simulink library "halout"  (R2021b)
settings: Solver=VariableStepAuto  StartTime=0.0  StopTime=10.0  RelTol=1e-3
undefined symbols (not defined in the file): C_TASK_5MS_S, FALSE, KHAL_CAN1TxReq_flg, KHAL_CAN2TxReq_flg, KHAL_CAN3FD3VCU1toNIDECTxReq_flg, KHAL_CAN3FD3VCU1TxReq_flg, KHAL_CAN3FD3VCU2E2E_flg, KHAL_CAN3FD3VCU2toNIDECE2E_flg, KHAL_CAN3FD3VCU2toNIDECTxReq_flg, KHAL_CAN3FD3VCU2TxReq_flg, KHAL_CAN3TxReq_flg, KHAL_CAN4FD4CE1000E2E_flg, KHAL_CAN4FD4CE1000TxReq_flg, KHAL_CAN4TxReq_flg, KHAL_CAN5TxReq_flg, KHAL_CAN7TxReq_flg, ONE_INT, TRUE, ZERO_INT
libraries: FVT_lib x258, simulink x115
(part 4 of 17)

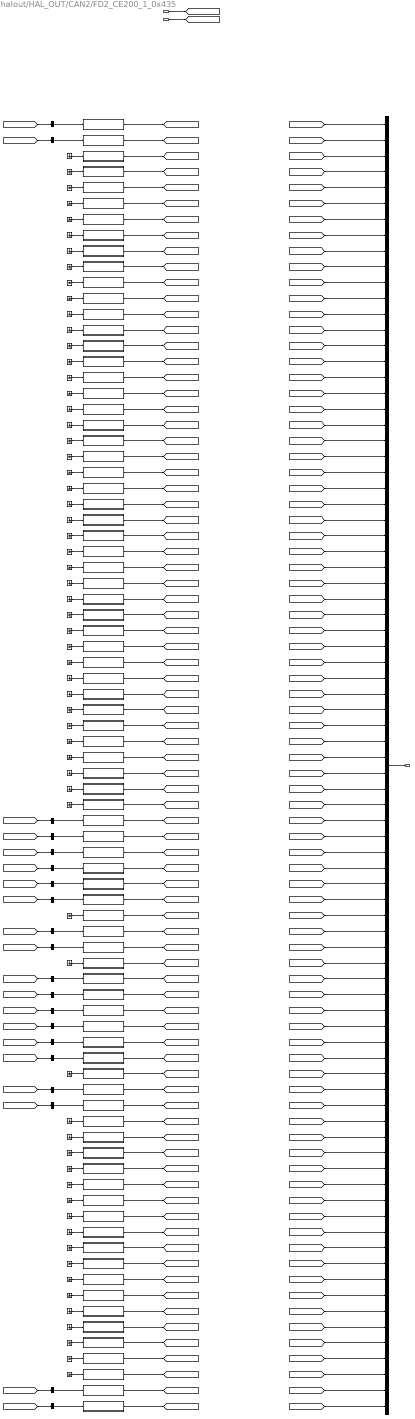
== system halout/HAL_OUT/CAN2/FD2_CE200_1_0x435 ==
  BSCP_outputs : Inport  OutDataTypeStr=Bus: BSCP_outputs
  BOUTP_outputs : Inport  Port=2  OutDataTypeStr=Bus: BOUTP_outputs
  AutoLTips : Subsystem
  CWheelTips : Subsystem
  FDCBCMAcc1StaSta : Subsystem
  FDCBCMAcc2StaSta : Subsystem
  FDCBCMAcc3StaSta : Subsystem
  FDCBCMAcc4StaSta : Subsystem
  FDCBCMAcc5StaSta : Subsystem
  FDCBCMAmbBrightStaSta : Subsystem
  FDCBCMAmbColorStaSta : Subsystem
  FDCBCMAmbDimENSta : Subsystem
  FDCBCMAmbFunENSta : Subsystem
  FDCBCMAmbLinkDriStaSta : Subsystem
  FDCBCMAmbODAENSta : Subsystem
  FDCBCMAmbPwrWarnENSta : Subsystem
  FDCBCMAmbWelENSta : Subsystem
  FDCBCMCLWinLockDrSta : Subsystem
  FDCBCMFollowMeENFunSta : Subsystem
  FDCBCMKey10AccSta : Subsystem
  FDCBCMKey1AccSta : Subsystem
  FDCBCMKey2AccSta : Subsystem
  FDCBCMKey3AccSta : Subsystem
  FDCBCMKey4AccSta : Subsystem
  FDCBCMKey5AccSta : Subsystem
  FDCBCMKey6AccSta : Subsystem
  FDCBCMKey7AccSta : Subsystem
  FDCBCMKey8AccSta : Subsystem
  FDCBCMKey9AccSta : Subsystem
  FDCBCMLockAlarmCmd : Subsystem
  FDCBCMPTGOpenHeightSta : Subsystem
  FDCBCMRmLpModeENFunSta : Subsystem
  FDCBCMTurnSwTSetStaSta : Subsystem
  FDCBCMUserNowSta : Subsystem
  FDCBCMWalkInUnLkEnFunSta : Subsystem
  FDCBCMWalkOutLkEnFunSta : Subsystem
  FDCDKCDkeyShowIVISta : Subsystem
  FDCDKCKeyMissSta : Subsystem
  FDCDKCKeyNumSta : Subsystem
  FDCDKCKeyTypeSta : Subsystem
  FDCDKCUIDLowPowerSta : Subsystem
  FDCSPTGSPTGENFunSta : Subsystem
  FDCTHCMAPTCForceOFFSta : Subsystem
  FDCTHCMAPTCWarningSta : Subsystem
  FDCTHCMAirIntZ3Sta : Subsystem
  Ground{,1..61} (62 alike) : Ground
  LFWheelShield : Subsystem
  LRBatWarn : Subsystem
  LRPressIndi : Subsystem
  LRSensorFail : Subsystem
  LRWheelDebug : Subsystem
  LRWheelPSW : Subsystem
  LRWheelPress : Subsystem
  LRWheelShield : Subsystem
  LRWheelTemp : Subsystem
  LRWheelTmpIndi : Subsystem
  RFWheelShield : Subsystem
  RRBatWarn : Subsystem
  RRPressIndi : Subsystem
  RRSensorFail : Subsystem
  RRWheelDebug : Subsystem
  RRWheelPSW : Subsystem
  RRWheelPress : Subsystem
  RRWheelShield : Subsystem
  RRWheelTemp : Subsystem
  RRWheelTmpIndi : Subsystem
  T1TPMSLFBatWarn : Subsystem
  T1TPMSLFPressIndi : Subsystem
  T1TPMSLFSensorFail : Subsystem
  T1TPMSLFWheelDebug : Subsystem
  T1TPMSLFWheelPSW : Subsystem
  T1TPMSLFWheelPress : Subsystem
  T1TPMSLFWheelTemp : Subsystem
  T1TPMSLFWheelTmpIndi : Subsystem
  T1TPMSRFBatWarn : Subsystem
  T1TPMSRFPressIndi : Subsystem
  T1TPMSRFSensorFail : Subsystem
  T1TPMSRFWheelDebug : Subsystem
  T1TPMSRFWheelPSW : Subsystem
  T1TPMSRFWheelPress : Subsystem
  T1TPMSRFWheelTemp : Subsystem
  T1TPMSRFWheelTmpIndi : Subsystem
  T1TPMSTPMSWarnIndi : Subsystem
  TPMSCaliButtAllow : Subsystem
  TPMSResButtAllow : Subsystem
  bus_creator : BusCreator  Inputs=82  OutDataTypeStr=Bus: DT_CAN2_SG_FD2_CE200_1  NonVirtualBus=on
  bus_selector : BusSelector  OutputSignals=VOUTP_AutoLTips_enum
  bus_selector1 : BusSelector  OutputSignals=VOUTP_CWheelTips_enum
  bus_selector10 : BusSelector  OutputSignals=VOUTP_RRBatWarn_flg
  bus_selector11 : BusSelector  OutputSignals=VOUTP_RRPressIndi_enum
  bus_selector12 : BusSelector  OutputSignals=VOUTP_RRSensorFail_flg
  bus_selector13 : BusSelector  OutputSignals=VOUTP_RRWheelDebug_flg
  bus_selector14 : BusSelector  OutputSignals=VOUTP_RRWheelPSW_raw8
  bus_selector15 : BusSelector  OutputSignals=VOUTP_RRWheelPress_raw8
  bus_selector16 : BusSelector  OutputSignals=VOUTP_RRWheelTemp_C
  bus_selector17 : BusSelector  OutputSignals=VOUTP_RRWheelTmpIndi_flg
  bus_selector18 : BusSelector  OutputSignals=VOUTP_TPMSCaliButtAllow_flg
  bus_selector19 : BusSelector  OutputSignals=VOUTP_TPMSResButtAllow_flg
  bus_selector2 : BusSelector  OutputSignals=VOUTP_LRBatWarn_flg
  bus_selector3 : BusSelector  OutputSignals=VOUTP_LRPressIndi_enum
  bus_selector4 : BusSelector  OutputSignals=VOUTP_LRSensorFail_flg
  bus_selector5 : BusSelector  OutputSignals=VOUTP_LRWheelDebug_flg
  bus_selector6 : BusSelector  OutputSignals=VOUTP_LRWheelPSW_raw8
  bus_selector7 : BusSelector  OutputSignals=VOUTP_LRWheelPress_raw8
  bus_selector8 : BusSelector  OutputSignals=VOUTP_LRWheelTemp_C
  bus_selector9 : BusSelector  OutputSignals=VOUTP_LRWheelTmpIndi_flg
  FD2_CE200_1 : Outport
  wires:
  BSCP_outputs/1 -> [BSCP_outputs]
  BOUTP_outputs/1 -> [BOUTP_outputs]
  [CAN2_AutoLTips] -> bus_creator/1  "CAN2_AutoLTips"
  [CAN2_CWheelTips] -> bus_creator/2  "CAN2_CWheelTips"
  [CAN2_FDC_BCM_Acc1Sta_Sta] -> bus_creator/3  "CAN2_FDC_BCM_Acc1Sta_Sta"
  [CAN2_FDC_BCM_Acc2Sta_Sta] -> bus_creator/4  "CAN2_FDC_BCM_Acc2Sta_Sta"
  [CAN2_FDC_BCM_Acc3Sta_Sta] -> bus_creator/5  "CAN2_FDC_BCM_Acc3Sta_Sta"
  [CAN2_FDC_BCM_Acc4Sta_Sta] -> bus_creator/6  "CAN2_FDC_BCM_Acc4Sta_Sta"
  [CAN2_FDC_BCM_Acc5Sta_Sta] -> bus_creator/7  "CAN2_FDC_BCM_Acc5Sta_Sta"
  [CAN2_FDC_BCM_AmbBrightSta_Sta] -> bus_creator/8  "CAN2_FDC_BCM_AmbBrightSta_Sta"
  [CAN2_FDC_BCM_AmbColorSta_Sta] -> bus_creator/9  "CAN2_FDC_BCM_AmbColorSta_Sta"
  [CAN2_FDC_BCM_AmbDimEN_Sta] -> bus_creator/10  "CAN2_FDC_BCM_AmbDimEN_Sta"
  [CAN2_FDC_BCM_AmbFunEN_Sta] -> bus_creator/11  "CAN2_FDC_BCM_AmbFunEN_Sta"
  [CAN2_FDC_BCM_AmbLinkDriSta_Sta] -> bus_creator/12  "CAN2_FDC_BCM_AmbLinkDriSta_Sta"
  [CAN2_FDC_BCM_AmbODAEN_Sta] -> bus_creator/13  "CAN2_FDC_BCM_AmbODAEN_Sta"
  [CAN2_FDC_BCM_AmbPwrWarnEN_Sta] -> bus_creator/14  "CAN2_FDC_BCM_AmbPwrWarnEN_Sta"
  [CAN2_FDC_BCM_AmbWelEN_Sta] -> bus_creator/15  "CAN2_FDC_BCM_AmbWelEN_Sta"
  [CAN2_FDC_BCM_CLWinLockDr_Sta] -> bus_creator/16  "CAN2_FDC_BCM_CLWinLockDr_Sta"
  [CAN2_FDC_BCM_FollowMeENFun_Sta] -> bus_creator/17  "CAN2_FDC_BCM_FollowMeENFun_Sta"
  [CAN2_FDC_BCM_Key10Acc_Sta] -> bus_creator/18  "CAN2_FDC_BCM_Key10Acc_Sta"
  [CAN2_FDC_BCM_Key1Acc_Sta] -> bus_creator/19  "CAN2_FDC_BCM_Key1Acc_Sta"
  [CAN2_FDC_BCM_Key2Acc_Sta] -> bus_creator/20  "CAN2_FDC_BCM_Key2Acc_Sta"
  [CAN2_FDC_BCM_Key3Acc_Sta] -> bus_creator/21  "CAN2_FDC_BCM_Key3Acc_Sta"
  [CAN2_FDC_BCM_Key4Acc_Sta] -> bus_creator/22  "CAN2_FDC_BCM_Key4Acc_Sta"
  [CAN2_FDC_BCM_Key5Acc_Sta] -> bus_creator/23  "CAN2_FDC_BCM_Key5Acc_Sta"
  [CAN2_FDC_BCM_Key6Acc_Sta] -> bus_creator/24  "CAN2_FDC_BCM_Key6Acc_Sta"
  [CAN2_FDC_BCM_Key7Acc_Sta] -> bus_creator/25  "CAN2_FDC_BCM_Key7Acc_Sta"
  [CAN2_FDC_BCM_Key8Acc_Sta] -> bus_creator/26  "CAN2_FDC_BCM_Key8Acc_Sta"
  [CAN2_FDC_BCM_Key9Acc_Sta] -> bus_creator/27  "CAN2_FDC_BCM_Key9Acc_Sta"
  [CAN2_FDC_BCM_LockAlarm_Cmd] -> bus_creator/28  "CAN2_FDC_BCM_LockAlarm_Cmd"
  [CAN2_FDC_BCM_PTGOpenHeight_Sta] -> bus_creator/29  "CAN2_FDC_BCM_PTGOpenHeight_Sta"
  [CAN2_FDC_BCM_RmLpModeENFun_Sta] -> bus_creator/30  "CAN2_FDC_BCM_RmLpModeENFun_Sta"
  [CAN2_FDC_BCM_TurnSwTSetSta_Sta] -> bus_creator/31  "CAN2_FDC_BCM_TurnSwTSetSta_Sta"
  [CAN2_FDC_BCM_UserNow_Sta] -> bus_creator/32  "CAN2_FDC_BCM_UserNow_Sta"
  [CAN2_FDC_BCM_WalkInUnLkEnFun_Sta] -> bus_creator/33  "CAN2_FDC_BCM_WalkInUnLkEnFun_Sta"
  [CAN2_FDC_BCM_WalkOutLkEnFun_Sta] -> bus_creator/34  "CAN2_FDC_BCM_WalkOutLkEnFun_Sta"
  [CAN2_FDC_DKC_DkeyShowIVI_Sta] -> bus_creator/35  "CAN2_FDC_DKC_DkeyShowIVI_Sta"
  [CAN2_FDC_DKC_KeyMiss_Sta] -> bus_creator/36  "CAN2_FDC_DKC_KeyMiss_Sta"
  [CAN2_FDC_DKC_KeyNum_Sta] -> bus_creator/37  "CAN2_FDC_DKC_KeyNum_Sta"
  [CAN2_FDC_DKC_KeyType_Sta] -> bus_creator/38  "CAN2_FDC_DKC_KeyType_Sta"
  [CAN2_FDC_DKC_UIDLowPower_Sta] -> bus_creator/39  "CAN2_FDC_DKC_UIDLowPower_Sta"
  [CAN2_FDC_SPTG_SPTGENFun_Sta] -> bus_creator/40  "CAN2_FDC_SPTG_SPTGENFun_Sta"
  [CAN2_FDC_THCM_APTCForceOFF_Sta] -> bus_creator/41  "CAN2_FDC_THCM_APTCForceOFF_Sta"
  [CAN2_FDC_THCM_APTCWarning_Sta] -> bus_creator/42  "CAN2_FDC_THCM_APTCWarning_Sta"
  [CAN2_FDC_THCM_AirIntZ3_Sta] -> bus_creator/43  "CAN2_FDC_THCM_AirIntZ3_Sta"
  [CAN2_LFWheelShield] -> bus_creator/44  "CAN2_LFWheelShield"
  [CAN2_LRBatWarn] -> bus_creator/45  "CAN2_LRBatWarn"
  [CAN2_LRPressIndi] -> bus_creator/46  "CAN2_LRPressIndi"
  [CAN2_LRSensorFail] -> bus_creator/47  "CAN2_LRSensorFail"
  [CAN2_LRWheelDebug] -> bus_creator/48  "CAN2_LRWheelDebug"
  [CAN2_LRWheelPSW] -> bus_creator/49  "CAN2_LRWheelPSW"
  [CAN2_LRWheelPress] -> bus_creator/50  "CAN2_LRWheelPress"
  [CAN2_LRWheelShield] -> bus_creator/51  "CAN2_LRWheelShield"
  [CAN2_LRWheelTemp] -> bus_creator/52  "CAN2_LRWheelTemp"
  [CAN2_LRWheelTmpIndi] -> bus_creator/53  "CAN2_LRWheelTmpIndi"
  [CAN2_RFWheelShield] -> bus_creator/54  "CAN2_RFWheelShield"
  [CAN2_RRBatWarn] -> bus_creator/55  "CAN2_RRBatWarn"
  [CAN2_RRPressIndi] -> bus_creator/56  "CAN2_RRPressIndi"
  [CAN2_RRSensorFail] -> bus_creator/57  "CAN2_RRSensorFail"
  [CAN2_RRWheelDebug] -> bus_creator/58  "CAN2_RRWheelDebug"
  [CAN2_RRWheelPSW] -> bus_creator/59  "CAN2_RRWheelPSW"
  [CAN2_RRWheelPress] -> bus_creator/60  "CAN2_RRWheelPress"
  [CAN2_RRWheelShield] -> bus_creator/61  "CAN2_RRWheelShield"
  [CAN2_RRWheelTemp] -> bus_creator/62  "CAN2_RRWheelTemp"
  [CAN2_RRWheelTmpIndi] -> bus_creator/63  "CAN2_RRWheelTmpIndi"
  [CAN2_T1_TPMS_LFBatWarn] -> bus_creator/64  "CAN2_T1_TPMS_LFBatWarn"
  [CAN2_T1_TPMS_LFPressIndi] -> bus_creator/65  "CAN2_T1_TPMS_LFPressIndi"
  [CAN2_T1_TPMS_LFSensorFail] -> bus_creator/66  "CAN2_T1_TPMS_LFSensorFail"
  [CAN2_T1_TPMS_LFWheelDebug] -> bus_creator/67  "CAN2_T1_TPMS_LFWheelDebug"
  [CAN2_T1_TPMS_LFWheelPSW] -> bus_creator/68  "CAN2_T1_TPMS_LFWheelPSW"
  [CAN2_T1_TPMS_LFWheelPress] -> bus_creator/69  "CAN2_T1_TPMS_LFWheelPress"
  [CAN2_T1_TPMS_LFWheelTemp] -> bus_creator/70  "CAN2_T1_TPMS_LFWheelTemp"
  [CAN2_T1_TPMS_LFWheelTmpIndi] -> bus_creator/71  "CAN2_T1_TPMS_LFWheelTmpIndi"
  [CAN2_T1_TPMS_RFBatWarn] -> bus_creator/72  "CAN2_T1_TPMS_RFBatWarn"
  [CAN2_T1_TPMS_RFPressIndi] -> bus_creator/73  "CAN2_T1_TPMS_RFPressIndi"
  [CAN2_T1_TPMS_RFSensorFail] -> bus_creator/74  "CAN2_T1_TPMS_RFSensorFail"
  [CAN2_T1_TPMS_RFWheelDebug] -> bus_creator/75  "CAN2_T1_TPMS_RFWheelDebug"
  [CAN2_T1_TPMS_RFWheelPSW] -> bus_creator/76  "CAN2_T1_TPMS_RFWheelPSW"
  [CAN2_T1_TPMS_RFWheelPress] -> bus_creator/77  "CAN2_T1_TPMS_RFWheelPress"
  [CAN2_T1_TPMS_RFWheelTemp] -> bus_creator/78  "CAN2_T1_TPMS_RFWheelTemp"
  [CAN2_T1_TPMS_RFWheelTmpIndi] -> bus_creator/79  "CAN2_T1_TPMS_RFWheelTmpIndi"
  [CAN2_T1_TPMS_TPMSWarnIndi] -> bus_creator/80  "CAN2_T1_TPMS_TPMSWarnIndi"
  [CAN2_TPMS_Cali_Butt_Allow] -> bus_creator/81  "CAN2_TPMS_Cali_Butt_Allow"
  [CAN2_TPMS_Res_Butt_Allow] -> bus_creator/82  "CAN2_TPMS_Res_Butt_Allow"
  bus_creator/1 -> FD2_CE200_1/1
  AutoLTips/1(CAN2_AutoLTips) -> [CAN2_AutoLTips]
  CWheelTips/1(CAN2_CWheelTips) -> [CAN2_CWheelTips]
  FDCBCMAcc1StaSta/1(CAN2_FDC_BCM_Acc1Sta_Sta) -> [CAN2_FDC_BCM_Acc1Sta_Sta]
  FDCBCMAcc2StaSta/1(CAN2_FDC_BCM_Acc2Sta_Sta) -> [CAN2_FDC_BCM_Acc2Sta_Sta]
  FDCBCMAcc3StaSta/1(CAN2_FDC_BCM_Acc3Sta_Sta) -> [CAN2_FDC_BCM_Acc3Sta_Sta]
  FDCBCMAcc4StaSta/1(CAN2_FDC_BCM_Acc4Sta_Sta) -> [CAN2_FDC_BCM_Acc4Sta_Sta]
  FDCBCMAcc5StaSta/1(CAN2_FDC_BCM_Acc5Sta_Sta) -> [CAN2_FDC_BCM_Acc5Sta_Sta]
  FDCBCMAmbBrightStaSta/1(CAN2_FDC_BCM_AmbBrightSta_Sta) -> [CAN2_FDC_BCM_AmbBrightSta_Sta]
  FDCBCMAmbColorStaSta/1(CAN2_FDC_BCM_AmbColorSta_Sta) -> [CAN2_FDC_BCM_AmbColorSta_Sta]
  FDCBCMAmbDimENSta/1(CAN2_FDC_BCM_AmbDimEN_Sta) -> [CAN2_FDC_BCM_AmbDimEN_Sta]
  FDCBCMAmbFunENSta/1(CAN2_FDC_BCM_AmbFunEN_Sta) -> [CAN2_FDC_BCM_AmbFunEN_Sta]
  FDCBCMAmbLinkDriStaSta/1(CAN2_FDC_BCM_AmbLinkDriSta_Sta) -> [CAN2_FDC_BCM_AmbLinkDriSta_Sta]
  FDCBCMAmbODAENSta/1(CAN2_FDC_BCM_AmbODAEN_Sta) -> [CAN2_FDC_BCM_AmbODAEN_Sta]
  FDCBCMAmbPwrWarnENSta/1(CAN2_FDC_BCM_AmbPwrWarnEN_Sta) -> [CAN2_FDC_BCM_AmbPwrWarnEN_Sta]
  FDCBCMAmbWelENSta/1(CAN2_FDC_BCM_AmbWelEN_Sta) -> [CAN2_FDC_BCM_AmbWelEN_Sta]
  FDCBCMCLWinLockDrSta/1(CAN2_FDC_BCM_CLWinLockDr_Sta) -> [CAN2_FDC_BCM_CLWinLockDr_Sta]
  FDCBCMFollowMeENFunSta/1(CAN2_FDC_BCM_FollowMeENFun_Sta) -> [CAN2_FDC_BCM_FollowMeENFun_Sta]
  FDCBCMKey10AccSta/1(CAN2_FDC_BCM_Key10Acc_Sta) -> [CAN2_FDC_BCM_Key10Acc_Sta]
  FDCBCMKey1AccSta/1(CAN2_FDC_BCM_Key1Acc_Sta) -> [CAN2_FDC_BCM_Key1Acc_Sta]
  FDCBCMKey2AccSta/1(CAN2_FDC_BCM_Key2Acc_Sta) -> [CAN2_FDC_BCM_Key2Acc_Sta]
  FDCBCMKey3AccSta/1(CAN2_FDC_BCM_Key3Acc_Sta) -> [CAN2_FDC_BCM_Key3Acc_Sta]
  FDCBCMKey4AccSta/1(CAN2_FDC_BCM_Key4Acc_Sta) -> [CAN2_FDC_BCM_Key4Acc_Sta]
  FDCBCMKey5AccSta/1(CAN2_FDC_BCM_Key5Acc_Sta) -> [CAN2_FDC_BCM_Key5Acc_Sta]
  FDCBCMKey6AccSta/1(CAN2_FDC_BCM_Key6Acc_Sta) -> [CAN2_FDC_BCM_Key6Acc_Sta]
  FDCBCMKey7AccSta/1(CAN2_FDC_BCM_Key7Acc_Sta) -> [CAN2_FDC_BCM_Key7Acc_Sta]
  FDCBCMKey8AccSta/1(CAN2_FDC_BCM_Key8Acc_Sta) -> [CAN2_FDC_BCM_Key8Acc_Sta]
  FDCBCMKey9AccSta/1(CAN2_FDC_BCM_Key9Acc_Sta) -> [CAN2_FDC_BCM_Key9Acc_Sta]
  FDCBCMLockAlarmCmd/1(CAN2_FDC_BCM_LockAlarm_Cmd) -> [CAN2_FDC_BCM_LockAlarm_Cmd]
  FDCBCMPTGOpenHeightSta/1(CAN2_FDC_BCM_PTGOpenHeight_Sta) -> [CAN2_FDC_BCM_PTGOpenHeight_Sta]
  FDCBCMRmLpModeENFunSta/1(CAN2_FDC_BCM_RmLpModeENFun_Sta) -> [CAN2_FDC_BCM_RmLpModeENFun_Sta]
  FDCBCMTurnSwTSetStaSta/1(CAN2_FDC_BCM_TurnSwTSetSta_Sta) -> [CAN2_FDC_BCM_TurnSwTSetSta_Sta]
  FDCBCMUserNowSta/1(CAN2_FDC_BCM_UserNow_Sta) -> [CAN2_FDC_BCM_UserNow_Sta]
  FDCBCMWalkInUnLkEnFunSta/1(CAN2_FDC_BCM_WalkInUnLkEnFun_Sta) -> [CAN2_FDC_BCM_WalkInUnLkEnFun_Sta]
  FDCBCMWalkOutLkEnFunSta/1(CAN2_FDC_BCM_WalkOutLkEnFun_Sta) -> [CAN2_FDC_BCM_WalkOutLkEnFun_Sta]
  FDCDKCDkeyShowIVISta/1(CAN2_FDC_DKC_DkeyShowIVI_Sta) -> [CAN2_FDC_DKC_DkeyShowIVI_Sta]
  FDCDKCKeyMissSta/1(CAN2_FDC_DKC_KeyMiss_Sta) -> [CAN2_FDC_DKC_KeyMiss_Sta]
  FDCDKCKeyNumSta/1(CAN2_FDC_DKC_KeyNum_Sta) -> [CAN2_FDC_DKC_KeyNum_Sta]
  FDCDKCKeyTypeSta/1(CAN2_FDC_DKC_KeyType_Sta) -> [CAN2_FDC_DKC_KeyType_Sta]
  FDCDKCUIDLowPowerSta/1(CAN2_FDC_DKC_UIDLowPower_Sta) -> [CAN2_FDC_DKC_UIDLowPower_Sta]
  FDCSPTGSPTGENFunSta/1(CAN2_FDC_SPTG_SPTGENFun_Sta) -> [CAN2_FDC_SPTG_SPTGENFun_Sta]
  FDCTHCMAPTCForceOFFSta/1(CAN2_FDC_THCM_APTCForceOFF_Sta) -> [CAN2_FDC_THCM_APTCForceOFF_Sta]
  FDCTHCMAPTCWarningSta/1(CAN2_FDC_THCM_APTCWarning_Sta) -> [CAN2_FDC_THCM_APTCWarning_Sta]
  FDCTHCMAirIntZ3Sta/1(CAN2_FDC_THCM_AirIntZ3_Sta) -> [CAN2_FDC_THCM_AirIntZ3_Sta]
  LFWheelShield/1(CAN2_LFWheelShield) -> [CAN2_LFWheelShield]
  LRBatWarn/1(CAN2_LRBatWarn) -> [CAN2_LRBatWarn]
  LRPressIndi/1(CAN2_LRPressIndi) -> [CAN2_LRPressIndi]
  LRSensorFail/1(CAN2_LRSensorFail) -> [CAN2_LRSensorFail]
  LRWheelDebug/1(CAN2_LRWheelDebug) -> [CAN2_LRWheelDebug]
  LRWheelPSW/1(CAN2_LRWheelPSW) -> [CAN2_LRWheelPSW]
  LRWheelPress/1(CAN2_LRWheelPress) -> [CAN2_LRWheelPress]
  LRWheelShield/1(CAN2_LRWheelShield) -> [CAN2_LRWheelShield]
  LRWheelTemp/1(CAN2_LRWheelTemp) -> [CAN2_LRWheelTemp]
  LRWheelTmpIndi/1(CAN2_LRWheelTmpIndi) -> [CAN2_LRWheelTmpIndi]
  RFWheelShield/1(CAN2_RFWheelShield) -> [CAN2_RFWheelShield]
  RRBatWarn/1(CAN2_RRBatWarn) -> [CAN2_RRBatWarn]
  RRPressIndi/1(CAN2_RRPressIndi) -> [CAN2_RRPressIndi]
  RRSensorFail/1(CAN2_RRSensorFail) -> [CAN2_RRSensorFail]
  RRWheelDebug/1(CAN2_RRWheelDebug) -> [CAN2_RRWheelDebug]
  RRWheelPSW/1(CAN2_RRWheelPSW) -> [CAN2_RRWheelPSW]
  RRWheelPress/1(CAN2_RRWheelPress) -> [CAN2_RRWheelPress]
  RRWheelShield/1(CAN2_RRWheelShield) -> [CAN2_RRWheelShield]
  RRWheelTemp/1(CAN2_RRWheelTemp) -> [CAN2_RRWheelTemp]
  RRWheelTmpIndi/1(CAN2_RRWheelTmpIndi) -> [CAN2_RRWheelTmpIndi]
  T1TPMSLFBatWarn/1(CAN2_T1_TPMS_LFBatWarn) -> [CAN2_T1_TPMS_LFBatWarn]
  T1TPMSLFPressIndi/1(CAN2_T1_TPMS_LFPressIndi) -> [CAN2_T1_TPMS_LFPressIndi]
  T1TPMSLFSensorFail/1(CAN2_T1_TPMS_LFSensorFail) -> [CAN2_T1_TPMS_LFSensorFail]
  T1TPMSLFWheelDebug/1(CAN2_T1_TPMS_LFWheelDebug) -> [CAN2_T1_TPMS_LFWheelDebug]
  T1TPMSLFWheelPSW/1(CAN2_T1_TPMS_LFWheelPSW) -> [CAN2_T1_TPMS_LFWheelPSW]
  T1TPMSLFWheelPress/1(CAN2_T1_TPMS_LFWheelPress) -> [CAN2_T1_TPMS_LFWheelPress]
  T1TPMSLFWheelTemp/1(CAN2_T1_TPMS_LFWheelTemp) -> [CAN2_T1_TPMS_LFWheelTemp]
  T1TPMSLFWheelTmpIndi/1(CAN2_T1_TPMS_LFWheelTmpIndi) -> [CAN2_T1_TPMS_LFWheelTmpIndi]
  T1TPMSRFBatWarn/1(CAN2_T1_TPMS_RFBatWarn) -> [CAN2_T1_TPMS_RFBatWarn]
  T1TPMSRFPressIndi/1(CAN2_T1_TPMS_RFPressIndi) -> [CAN2_T1_TPMS_RFPressIndi]
  T1TPMSRFSensorFail/1(CAN2_T1_TPMS_RFSensorFail) -> [CAN2_T1_TPMS_RFSensorFail]
  T1TPMSRFWheelDebug/1(CAN2_T1_TPMS_RFWheelDebug) -> [CAN2_T1_TPMS_RFWheelDebug]
  T1TPMSRFWheelPSW/1(CAN2_T1_TPMS_RFWheelPSW) -> [CAN2_T1_TPMS_RFWheelPSW]
  T1TPMSRFWheelPress/1(CAN2_T1_TPMS_RFWheelPress) -> [CAN2_T1_TPMS_RFWheelPress]
  T1TPMSRFWheelTemp/1(CAN2_T1_TPMS_RFWheelTemp) -> [CAN2_T1_TPMS_RFWheelTemp]
  T1TPMSRFWheelTmpIndi/1(CAN2_T1_TPMS_RFWheelTmpIndi) -> [CAN2_T1_TPMS_RFWheelTmpIndi]
  T1TPMSTPMSWarnIndi/1(CAN2_T1_TPMS_TPMSWarnIndi) -> [CAN2_T1_TPMS_TPMSWarnIndi]
  TPMSCaliButtAllow/1(CAN2_TPMS_Cali_Butt_Allow) -> [CAN2_TPMS_Cali_Butt_Allow]
  TPMSResButtAllow/1(CAN2_TPMS_Res_Butt_Allow) -> [CAN2_TPMS_Res_Butt_Allow]
  bus_selector/1 -> AutoLTips/1(AutoLTips)  "<VOUTP_AutoLTips_enum>"
  [BOUTP_outputs] -> bus_selector/1
  bus_selector1/1 -> CWheelTips/1(CWheelTips)  "<VOUTP_CWheelTips_enum>"
  [BOUTP_outputs] -> bus_selector1/1
  Ground/1 -> FDCBCMAcc1StaSta/1(FDCBCMAcc1StaSta)
  Ground1/1 -> FDCBCMAcc2StaSta/1(FDCBCMAcc2StaSta)
  Ground2/1 -> FDCBCMAcc3StaSta/1(FDCBCMAcc3StaSta)
  Ground3/1 -> FDCBCMAcc4StaSta/1(FDCBCMAcc4StaSta)
  Ground4/1 -> FDCBCMAcc5StaSta/1(FDCBCMAcc5StaSta)
  Ground5/1 -> FDCBCMAmbBrightStaSta/1(FDCBCMAmbBrightStaSta)
  Ground6/1 -> FDCBCMAmbColorStaSta/1(FDCBCMAmbColorStaSta)
  Ground7/1 -> FDCBCMAmbDimENSta/1(FDCBCMAmbDimENSta)
  Ground8/1 -> FDCBCMAmbFunENSta/1(FDCBCMAmbFunENSta)
  Ground9/1 -> FDCBCMAmbLinkDriStaSta/1(FDCBCMAmbLinkDriStaSta)
  Ground10/1 -> FDCBCMAmbODAENSta/1(FDCBCMAmbODAENSta)
  Ground11/1 -> FDCBCMAmbPwrWarnENSta/1(FDCBCMAmbPwrWarnENSta)
  Ground12/1 -> FDCBCMAmbWelENSta/1(FDCBCMAmbWelENSta)
  Ground13/1 -> FDCBCMCLWinLockDrSta/1(FDCBCMCLWinLockDrSta)
  Ground14/1 -> FDCBCMFollowMeENFunSta/1(FDCBCMFollowMeENFunSta)
  Ground15/1 -> FDCBCMKey10AccSta/1(FDCBCMKey10AccSta)
  Ground16/1 -> FDCBCMKey1AccSta/1(FDCBCMKey1AccSta)
  Ground17/1 -> FDCBCMKey2AccSta/1(FDCBCMKey2AccSta)
  Ground18/1 -> FDCBCMKey3AccSta/1(FDCBCMKey3AccSta)
  Ground19/1 -> FDCBCMKey4AccSta/1(FDCBCMKey4AccSta)
  Ground20/1 -> FDCBCMKey5AccSta/1(FDCBCMKey5AccSta)
  Ground21/1 -> FDCBCMKey6AccSta/1(FDCBCMKey6AccSta)
  Ground22/1 -> FDCBCMKey7AccSta/1(FDCBCMKey7AccSta)
  Ground23/1 -> FDCBCMKey8AccSta/1(FDCBCMKey8AccSta)
  Ground24/1 -> FDCBCMKey9AccSta/1(FDCBCMKey9AccSta)
  Ground25/1 -> FDCBCMLockAlarmCmd/1(FDCBCMLockAlarmCmd)
  Ground26/1 -> FDCBCMPTGOpenHeightSta/1(FDCBCMPTGOpenHeightSta)
  Ground27/1 -> FDCBCMRmLpModeENFunSta/1(FDCBCMRmLpModeENFunSta)
  Ground28/1 -> FDCBCMTurnSwTSetStaSta/1(FDCBCMTurnSwTSetStaSta)
  Ground29/1 -> FDCBCMUserNowSta/1(FDCBCMUserNowSta)
  Ground30/1 -> FDCBCMWalkInUnLkEnFunSta/1(FDCBCMWalkInUnLkEnFunSta)
  Ground31/1 -> FDCBCMWalkOutLkEnFunSta/1(FDCBCMWalkOutLkEnFunSta)
  Ground32/1 -> FDCDKCDkeyShowIVISta/1(FDCDKCDkeyShowIVISta)
  Ground33/1 -> FDCDKCKeyMissSta/1(FDCDKCKeyMissSta)
  Ground34/1 -> FDCDKCKeyNumSta/1(FDCDKCKeyNumSta)
  Ground35/1 -> FDCDKCKeyTypeSta/1(FDCDKCKeyTypeSta)
  Ground36/1 -> FDCDKCUIDLowPowerSta/1(FDCDKCUIDLowPowerSta)
  Ground37/1 -> FDCSPTGSPTGENFunSta/1(FDCSPTGSPTGENFunSta)
  Ground38/1 -> FDCTHCMAPTCForceOFFSta/1(FDCTHCMAPTCForceOFFSta)
  Ground39/1 -> FDCTHCMAPTCWarningSta/1(FDCTHCMAPTCWarningSta)
  Ground40/1 -> FDCTHCMAirIntZ3Sta/1(FDCTHCMAirIntZ3Sta)
  Ground41/1 -> LFWheelShield/1(LFWheelShield)
  bus_selector2/1 -> LRBatWarn/1(LRBatWarn)  "<VOUTP_LRBatWarn_flg>"
  [BOUTP_outputs] -> bus_selector2/1
  bus_selector3/1 -> LRPressIndi/1(LRPressIndi)  "<VOUTP_LRPressIndi_enum>"
  [BOUTP_outputs] -> bus_selector3/1
  bus_selector4/1 -> LRSensorFail/1(LRSensorFail)  "<VOUTP_LRSensorFail_flg>"
  [BOUTP_outputs] -> bus_selector4/1
  bus_selector5/1 -> LRWheelDebug/1(LRWheelDebug)  "<VOUTP_LRWheelDebug_flg>"
  [BOUTP_outputs] -> bus_selector5/1
  bus_selector6/1 -> LRWheelPSW/1(LRWheelPSW)  "<VOUTP_LRWheelPSW_raw8>"
  [BOUTP_outputs] -> bus_selector6/1
  bus_selector7/1 -> LRWheelPress/1(LRWheelPress)  "<VOUTP_LRWheelPress_raw8>"
  [BOUTP_outputs] -> bus_selector7/1
  Ground42/1 -> LRWheelShield/1(LRWheelShield)
  bus_selector8/1 -> LRWheelTemp/1(LRWheelTemp)  "<VOUTP_LRWheelTemp_C>"
  [BOUTP_outputs] -> bus_selector8/1
  bus_selector9/1 -> LRWheelTmpIndi/1(LRWheelTmpIndi)  "<VOUTP_LRWheelTmpIndi_flg>"
  [BOUTP_outputs] -> bus_selector9/1
  Ground43/1 -> RFWheelShield/1(RFWheelShield)
  bus_selector10/1 -> RRBatWarn/1(RRBatWarn)  "<VOUTP_RRBatWarn_flg>"
  [BOUTP_outputs] -> bus_selector10/1
  bus_selector11/1 -> RRPressIndi/1(RRPressIndi)  "<VOUTP_RRPressIndi_enum>"
  [BOUTP_outputs] -> bus_selector11/1
  bus_selector12/1 -> RRSensorFail/1(RRSensorFail)  "<VOUTP_RRSensorFail_flg>"
  [BOUTP_outputs] -> bus_selector12/1
  bus_selector13/1 -> RRWheelDebug/1(RRWheelDebug)  "<VOUTP_RRWheelDebug_flg>"
  [BOUTP_outputs] -> bus_selector13/1
  bus_selector14/1 -> RRWheelPSW/1(RRWheelPSW)  "<VOUTP_RRWheelPSW_raw8>"
  [BOUTP_outputs] -> bus_selector14/1
  bus_selector15/1 -> RRWheelPress/1(RRWheelPress)  "<VOUTP_RRWheelPress_raw8>"
  [BOUTP_outputs] -> bus_selector15/1
  Ground44/1 -> RRWheelShield/1(RRWheelShield)
  bus_selector16/1 -> RRWheelTemp/1(RRWheelTemp)  "<VOUTP_RRWheelTemp_C>"
  [BOUTP_outputs] -> bus_selector16/1
  bus_selector17/1 -> RRWheelTmpIndi/1(RRWheelTmpIndi)  "<VOUTP_RRWheelTmpIndi_flg>"
  [BOUTP_outputs] -> bus_selector17/1
  Ground45/1 -> T1TPMSLFBatWarn/1(T1TPMSLFBatWarn)
  Ground46/1 -> T1TPMSLFPressIndi/1(T1TPMSLFPressIndi)
  Ground47/1 -> T1TPMSLFSensorFail/1(T1TPMSLFSensorFail)
  Ground48/1 -> T1TPMSLFWheelDebug/1(T1TPMSLFWheelDebug)
  Ground49/1 -> T1TPMSLFWheelPSW/1(T1TPMSLFWheelPSW)
  Ground50/1 -> T1TPMSLFWheelPress/1(T1TPMSLFWheelPress)
  Ground51/1 -> T1TPMSLFWheelTemp/1(T1TPMSLFWheelTemp)
  Ground52/1 -> T1TPMSLFWheelTmpIndi/1(T1TPMSLFWheelTmpIndi)
  Ground53/1 -> T1TPMSRFBatWarn/1(T1TPMSRFBatWarn)
  Ground54/1 -> T1TPMSRFPressIndi/1(T1TPMSRFPressIndi)
  Ground55/1 -> T1TPMSRFSensorFail/1(T1TPMSRFSensorFail)
  Ground56/1 -> T1TPMSRFWheelDebug/1(T1TPMSRFWheelDebug)
  Ground57/1 -> T1TPMSRFWheelPSW/1(T1TPMSRFWheelPSW)
  Ground58/1 -> T1TPMSRFWheelPress/1(T1TPMSRFWheelPress)
  Ground59/1 -> T1TPMSRFWheelTemp/1(T1TPMSRFWheelTemp)
  Ground60/1 -> T1TPMSRFWheelTmpIndi/1(T1TPMSRFWheelTmpIndi)
  Ground61/1 -> T1TPMSTPMSWarnIndi/1(T1TPMSTPMSWarnIndi)
  bus_selector18/1 -> TPMSCaliButtAllow/1(TPMSCaliButtAllow)  "<VOUTP_TPMSCaliButtAllow_flg>"
  [BOUTP_outputs] -> bus_selector18/1
  bus_selector19/1 -> TPMSResButtAllow/1(TPMSResButtAllow)  "<VOUTP_TPMSResButtAllow_flg>"
  [BOUTP_outputs] -> bus_selector19/1

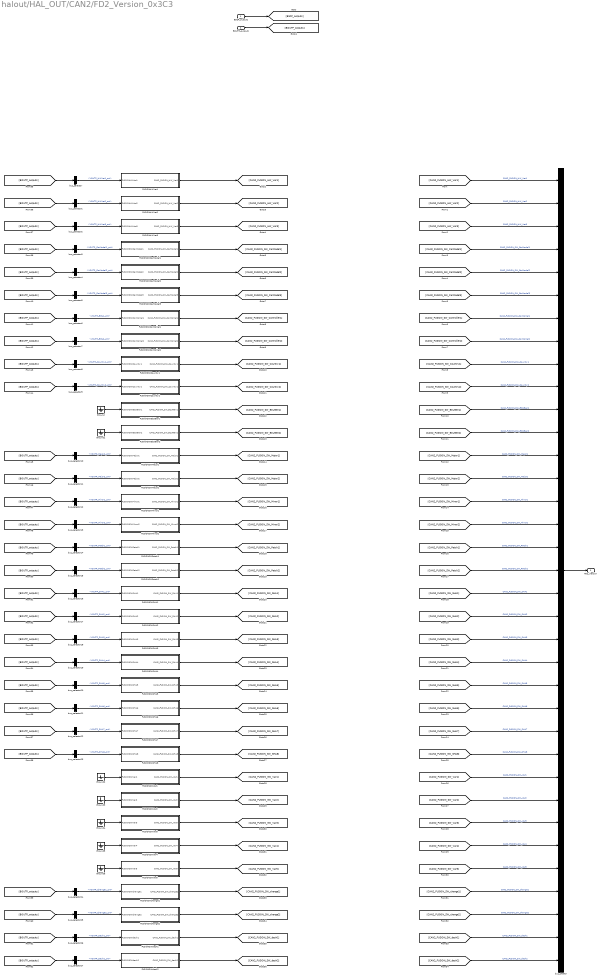
== system halout/HAL_OUT/CAN2/FD2_Version_0x3C3 ==
  BSCP_outputs : Inport  OutDataTypeStr=Bus: BSCP_outputs
  BOUTP_outputs : Inport  Port=2  OutDataTypeStr=Bus: BOUTP_outputs
  FUSIONHWVer1 : Subsystem
  FUSIONHWVer2 : Subsystem
  FUSIONHWVer3 : Subsystem
  FUSIONSWCarModel1 : Subsystem
  FUSIONSWCarModel2 : Subsystem
  FUSIONSWCarModel3 : Subsystem
  FUSIONSWController1 : Subsystem
  FUSIONSWController2 : Subsystem
  FUSIONSWCountry1 : Subsystem
  FUSIONSWCountry2 : Subsystem
  FUSIONSWECUGen1 : Subsystem
  FUSIONSWECUGen2 : Subsystem
  FUSIONSWMajor1 : Subsystem
  FUSIONSWMajor2 : Subsystem
  FUSIONSWMinor1 : Subsystem
  FUSIONSWMinor2 : Subsystem
  FUSIONSWPatch1 : Subsystem
  FUSIONSWPatch2 : Subsystem
  FUSIONSWSHA1 : Subsystem
  FUSIONSWSHA2 : Subsystem
  FUSIONSWSHA3 : Subsystem
  FUSIONSWSHA4 : Subsystem
  FUSIONSWSHA5 : Subsystem
  FUSIONSWSHA6 : Subsystem
  FUSIONSWSHA7 : Subsystem
  FUSIONSWSHA8 : Subsystem
  FUSIONSWVar1 : Subsystem
  FUSIONSWVar2 : Subsystem
  FUSIONSWVar3 : Subsystem
  FUSIONSWVar4 : Subsystem
  FUSIONSWVar5 : Subsystem
  FUSIONSWchange1 : Subsystem
  FUSIONSWchange2 : Subsystem
  FUSIONSWdash1 : Subsystem
  FUSIONSWdash2 : Subsystem
  Ground{,1..6} (7 alike) : Ground
  bus_creator : BusCreator  Inputs=35  OutDataTypeStr=Bus: DT_CAN2_SG_FD2_Version  NonVirtualBus=on
  bus_selector : BusSelector  OutputSignals=VOUTP_HWVer1_cnt
  bus_selector1 : BusSelector  OutputSignals=VOUTP_HWVer2_cnt
  bus_selector10 : BusSelector  OutputSignals=VOUTP_Major1_cnt
  bus_selector11 : BusSelector  OutputSignals=VOUTP_Major2_cnt
  bus_selector12 : BusSelector  OutputSignals=VOUTP_Minor1_cnt
  bus_selector13 : BusSelector  OutputSignals=VOUTP_Minor2_cnt
  bus_selector14 : BusSelector  OutputSignals=VOUTP_Patch1_cnt
  bus_selector15 : BusSelector  OutputSignals=VOUTP_Patch2_cnt
  bus_selector16 : BusSelector  OutputSignals=VOUTP_SHA1_cnt
  bus_selector17 : BusSelector  OutputSignals=VOUTP_SHA2_cnt
  bus_selector18 : BusSelector  OutputSignals=VOUTP_SHA3_cnt
  bus_selector19 : BusSelector  OutputSignals=VOUTP_SHA4_cnt
  bus_selector2 : BusSelector  OutputSignals=VOUTP_HWVer3_cnt
  bus_selector20 : BusSelector  OutputSignals=VOUTP_SHA5_cnt
  bus_selector21 : BusSelector  OutputSignals=VOUTP_SHA6_cnt
  bus_selector22 : BusSelector  OutputSignals=VOUTP_SHA7_cnt
  bus_selector23 : BusSelector  OutputSignals=VOUTP_SHA8_cnt
  bus_selector24 : BusSelector  OutputSignals=VOUTP_Change1_cnt
  bus_selector25 : BusSelector  OutputSignals=VOUTP_Change2_cnt
  bus_selector26 : BusSelector  OutputSignals=VOUTP_Dash1_cnt
  bus_selector27 : BusSelector  OutputSignals=VOUTP_Dash2_cnt
  bus_selector3 : BusSelector  OutputSignals=VOUTP_CarModel1_cnt
  bus_selector4 : BusSelector  OutputSignals=VOUTP_CarModel2_cnt
  bus_selector5 : BusSelector  OutputSignals=VOUTP_CarModel3_cnt
  bus_selector6 : BusSelector  OutputSignals=VOUTP_ECU1_cnt
  bus_selector7 : BusSelector  OutputSignals=VOUTP_ECU2_cnt
  bus_selector8 : BusSelector  OutputSignals=VOUTP_Country1_cnt
  bus_selector9 : BusSelector  OutputSignals=VOUTP_Country2_cnt
  FD2_Version : Outport
  wires:
  BSCP_outputs/1 -> [BSCP_outputs]
  BOUTP_outputs/1 -> [BOUTP_outputs]
  [CAN2_FUSION_HW_Ver1] -> bus_creator/1  "CAN2_FUSION_HW_Ver1"
  [CAN2_FUSION_HW_Ver2] -> bus_creator/2  "CAN2_FUSION_HW_Ver2"
  [CAN2_FUSION_HW_Ver3] -> bus_creator/3  "CAN2_FUSION_HW_Ver3"
  [CAN2_FUSION_SW_CarModel1] -> bus_creator/4  "CAN2_FUSION_SW_CarModel1"
  [CAN2_FUSION_SW_CarModel2] -> bus_creator/5  "CAN2_FUSION_SW_CarModel2"
  [CAN2_FUSION_SW_CarModel3] -> bus_creator/6  "CAN2_FUSION_SW_CarModel3"
  [CAN2_FUSION_SW_Controller1] -> bus_creator/7  "CAN2_FUSION_SW_Controller1"
  [CAN2_FUSION_SW_Controller2] -> bus_creator/8  "CAN2_FUSION_SW_Controller2"
  [CAN2_FUSION_SW_Country1] -> bus_creator/9  "CAN2_FUSION_SW_Country1"
  [CAN2_FUSION_SW_Country2] -> bus_creator/10  "CAN2_FUSION_SW_Country2"
  [CAN2_FUSION_SW_ECUGen1] -> bus_creator/11  "CAN2_FUSION_SW_ECUGen1"
  [CAN2_FUSION_SW_ECUGen2] -> bus_creator/12  "CAN2_FUSION_SW_ECUGen2"
  [CAN2_FUSION_SW_Major1] -> bus_creator/13  "CAN2_FUSION_SW_Major1"
  [CAN2_FUSION_SW_Major2] -> bus_creator/14  "CAN2_FUSION_SW_Major2"
  [CAN2_FUSION_SW_Minor1] -> bus_creator/15  "CAN2_FUSION_SW_Minor1"
  [CAN2_FUSION_SW_Minor2] -> bus_creator/16  "CAN2_FUSION_SW_Minor2"
  [CAN2_FUSION_SW_Patch1] -> bus_creator/17  "CAN2_FUSION_SW_Patch1"
  [CAN2_FUSION_SW_Patch2] -> bus_creator/18  "CAN2_FUSION_SW_Patch2"
  [CAN2_FUSION_SW_SHA1] -> bus_creator/19  "CAN2_FUSION_SW_SHA1"
  [CAN2_FUSION_SW_SHA2] -> bus_creator/20  "CAN2_FUSION_SW_SHA2"
  [CAN2_FUSION_SW_SHA3] -> bus_creator/21  "CAN2_FUSION_SW_SHA3"
  [CAN2_FUSION_SW_SHA4] -> bus_creator/22  "CAN2_FUSION_SW_SHA4"
  [CAN2_FUSION_SW_SHA5] -> bus_creator/23  "CAN2_FUSION_SW_SHA5"
  [CAN2_FUSION_SW_SHA6] -> bus_creator/24  "CAN2_FUSION_SW_SHA6"
  [CAN2_FUSION_SW_SHA7] -> bus_creator/25  "CAN2_FUSION_SW_SHA7"
  [CAN2_FUSION_SW_SHA8] -> bus_creator/26  "CAN2_FUSION_SW_SHA8"
  [CAN2_FUSION_SW_Var1] -> bus_creator/27  "CAN2_FUSION_SW_Var1"
  [CAN2_FUSION_SW_Var2] -> bus_creator/28  "CAN2_FUSION_SW_Var2"
  [CAN2_FUSION_SW_Var3] -> bus_creator/29  "CAN2_FUSION_SW_Var3"
  [CAN2_FUSION_SW_Var4] -> bus_creator/30  "CAN2_FUSION_SW_Var4"
  [CAN2_FUSION_SW_Var5] -> bus_creator/31  "CAN2_FUSION_SW_Var5"
  [CAN2_FUSION_SW_change1] -> bus_creator/32  "CAN2_FUSION_SW_change1"
  [CAN2_FUSION_SW_change2] -> bus_creator/33  "CAN2_FUSION_SW_change2"
  [CAN2_FUSION_SW_dash1] -> bus_creator/34  "CAN2_FUSION_SW_dash1"
  [CAN2_FUSION_SW_dash2] -> bus_creator/35  "CAN2_FUSION_SW_dash2"
  bus_creator/1 -> FD2_Version/1
  FUSIONHWVer1/1(CAN2_FUSION_HW_Ver1) -> [CAN2_FUSION_HW_Ver1]
  FUSIONHWVer2/1(CAN2_FUSION_HW_Ver2) -> [CAN2_FUSION_HW_Ver2]
  FUSIONHWVer3/1(CAN2_FUSION_HW_Ver3) -> [CAN2_FUSION_HW_Ver3]
  FUSIONSWCarModel1/1(CAN2_FUSION_SW_CarModel1) -> [CAN2_FUSION_SW_CarModel1]
  FUSIONSWCarModel2/1(CAN2_FUSION_SW_CarModel2) -> [CAN2_FUSION_SW_CarModel2]
  FUSIONSWCarModel3/1(CAN2_FUSION_SW_CarModel3) -> [CAN2_FUSION_SW_CarModel3]
  FUSIONSWController1/1(CAN2_FUSION_SW_Controller1) -> [CAN2_FUSION_SW_Controller1]
  FUSIONSWController2/1(CAN2_FUSION_SW_Controller2) -> [CAN2_FUSION_SW_Controller2]
  FUSIONSWCountry1/1(CAN2_FUSION_SW_Country1) -> [CAN2_FUSION_SW_Country1]
  FUSIONSWCountry2/1(CAN2_FUSION_SW_Country2) -> [CAN2_FUSION_SW_Country2]
  FUSIONSWECUGen1/1(CAN2_FUSION_SW_ECUGen1) -> [CAN2_FUSION_SW_ECUGen1]
  FUSIONSWECUGen2/1(CAN2_FUSION_SW_ECUGen2) -> [CAN2_FUSION_SW_ECUGen2]
  FUSIONSWMajor1/1(CAN2_FUSION_SW_Major1) -> [CAN2_FUSION_SW_Major1]
  FUSIONSWMajor2/1(CAN2_FUSION_SW_Major2) -> [CAN2_FUSION_SW_Major2]
  FUSIONSWMinor1/1(CAN2_FUSION_SW_Minor1) -> [CAN2_FUSION_SW_Minor1]
  FUSIONSWMinor2/1(CAN2_FUSION_SW_Minor2) -> [CAN2_FUSION_SW_Minor2]
  FUSIONSWPatch1/1(CAN2_FUSION_SW_Patch1) -> [CAN2_FUSION_SW_Patch1]
  FUSIONSWPatch2/1(CAN2_FUSION_SW_Patch2) -> [CAN2_FUSION_SW_Patch2]
  FUSIONSWSHA1/1(CAN2_FUSION_SW_SHA1) -> [CAN2_FUSION_SW_SHA1]
  FUSIONSWSHA2/1(CAN2_FUSION_SW_SHA2) -> [CAN2_FUSION_SW_SHA2]
  FUSIONSWSHA3/1(CAN2_FUSION_SW_SHA3) -> [CAN2_FUSION_SW_SHA3]
  FUSIONSWSHA4/1(CAN2_FUSION_SW_SHA4) -> [CAN2_FUSION_SW_SHA4]
  FUSIONSWSHA5/1(CAN2_FUSION_SW_SHA5) -> [CAN2_FUSION_SW_SHA5]
  FUSIONSWSHA6/1(CAN2_FUSION_SW_SHA6) -> [CAN2_FUSION_SW_SHA6]
  FUSIONSWSHA7/1(CAN2_FUSION_SW_SHA7) -> [CAN2_FUSION_SW_SHA7]
  FUSIONSWSHA8/1(CAN2_FUSION_SW_SHA8) -> [CAN2_FUSION_SW_SHA8]
  FUSIONSWVar1/1(CAN2_FUSION_SW_Var1) -> [CAN2_FUSION_SW_Var1]
  FUSIONSWVar2/1(CAN2_FUSION_SW_Var2) -> [CAN2_FUSION_SW_Var2]
  FUSIONSWVar3/1(CAN2_FUSION_SW_Var3) -> [CAN2_FUSION_SW_Var3]
  FUSIONSWVar4/1(CAN2_FUSION_SW_Var4) -> [CAN2_FUSION_SW_Var4]
  FUSIONSWVar5/1(CAN2_FUSION_SW_Var5) -> [CAN2_FUSION_SW_Var5]
  FUSIONSWchange1/1(CAN2_FUSION_SW_change1) -> [CAN2_FUSION_SW_change1]
  FUSIONSWchange2/1(CAN2_FUSION_SW_change2) -> [CAN2_FUSION_SW_change2]
  FUSIONSWdash1/1(CAN2_FUSION_SW_dash1) -> [CAN2_FUSION_SW_dash1]
  FUSIONSWdash2/1(CAN2_FUSION_SW_dash2) -> [CAN2_FUSION_SW_dash2]
  bus_selector/1 -> FUSIONHWVer1/1(FUSIONHWVer1)  "<VOUTP_HWVer1_cnt>"
  [BOUTP_outputs] -> bus_selector/1
  bus_selector1/1 -> FUSIONHWVer2/1(FUSIONHWVer2)  "<VOUTP_HWVer2_cnt>"
  [BOUTP_outputs] -> bus_selector1/1
  bus_selector2/1 -> FUSIONHWVer3/1(FUSIONHWVer3)  "<VOUTP_HWVer3_cnt>"
  [BOUTP_outputs] -> bus_selector2/1
  bus_selector3/1 -> FUSIONSWCarModel1/1(FUSIONSWCarModel1)  "<VOUTP_CarModel1_cnt>"
  [BOUTP_outputs] -> bus_selector3/1
  bus_selector4/1 -> FUSIONSWCarModel2/1(FUSIONSWCarModel2)  "<VOUTP_CarModel2_cnt>"
  [BOUTP_outputs] -> bus_selector4/1
  bus_selector5/1 -> FUSIONSWCarModel3/1(FUSIONSWCarModel3)  "<VOUTP_CarModel3_cnt>"
  [BOUTP_outputs] -> bus_selector5/1
  bus_selector6/1 -> FUSIONSWController1/1(FUSIONSWController1)  "<VOUTP_ECU1_cnt>"
  [BOUTP_outputs] -> bus_selector6/1
  bus_selector7/1 -> FUSIONSWController2/1(FUSIONSWController2)  "<VOUTP_ECU2_cnt>"
  [BOUTP_outputs] -> bus_selector7/1
  bus_selector8/1 -> FUSIONSWCountry1/1(FUSIONSWCountry1)  "<VOUTP_Country1_cnt>"
  [BOUTP_outputs] -> bus_selector8/1
  bus_selector9/1 -> FUSIONSWCountry2/1(FUSIONSWCountry2)  "<VOUTP_Country2_cnt>"
  [BOUTP_outputs] -> bus_selector9/1
  Ground/1 -> FUSIONSWECUGen1/1(FUSIONSWECUGen1)
  Ground1/1 -> FUSIONSWECUGen2/1(FUSIONSWECUGen2)
  bus_selector10/1 -> FUSIONSWMajor1/1(FUSIONSWMajor1)  "<VOUTP_Major1_cnt>"
  [BOUTP_outputs] -> bus_selector10/1
  bus_selector11/1 -> FUSIONSWMajor2/1(FUSIONSWMajor2)  "<VOUTP_Major2_cnt>"
  [BOUTP_outputs] -> bus_selector11/1
  bus_selector12/1 -> FUSIONSWMinor1/1(FUSIONSWMinor1)  "<VOUTP_Minor1_cnt>"
  [BOUTP_outputs] -> bus_selector12/1
  bus_selector13/1 -> FUSIONSWMinor2/1(FUSIONSWMinor2)  "<VOUTP_Minor2_cnt>"
  [BOUTP_outputs] -> bus_selector13/1
  bus_selector14/1 -> FUSIONSWPatch1/1(FUSIONSWPatch1)  "<VOUTP_Patch1_cnt>"
  [BOUTP_outputs] -> bus_selector14/1
  bus_selector15/1 -> FUSIONSWPatch2/1(FUSIONSWPatch2)  "<VOUTP_Patch2_cnt>"
  [BOUTP_outputs] -> bus_selector15/1
  bus_selector16/1 -> FUSIONSWSHA1/1(FUSIONSWSHA1)  "<VOUTP_SHA1_cnt>"
  [BOUTP_outputs] -> bus_selector16/1
  bus_selector17/1 -> FUSIONSWSHA2/1(FUSIONSWSHA2)  "<VOUTP_SHA2_cnt>"
  [BOUTP_outputs] -> bus_selector17/1
  bus_selector18/1 -> FUSIONSWSHA3/1(FUSIONSWSHA3)  "<VOUTP_SHA3_cnt>"
  [BOUTP_outputs] -> bus_selector18/1
  bus_selector19/1 -> FUSIONSWSHA4/1(FUSIONSWSHA4)  "<VOUTP_SHA4_cnt>"
  [BOUTP_outputs] -> bus_selector19/1
  bus_selector20/1 -> FUSIONSWSHA5/1(FUSIONSWSHA5)  "<VOUTP_SHA5_cnt>"
  [BOUTP_outputs] -> bus_selector20/1
  bus_selector21/1 -> FUSIONSWSHA6/1(FUSIONSWSHA6)  "<VOUTP_SHA6_cnt>"
  [BOUTP_outputs] -> bus_selector21/1
  bus_selector22/1 -> FUSIONSWSHA7/1(FUSIONSWSHA7)  "<VOUTP_SHA7_cnt>"
  [BOUTP_outputs] -> bus_selector22/1
  bus_selector23/1 -> FUSIONSWSHA8/1(FUSIONSWSHA8)  "<VOUTP_SHA8_cnt>"
  [BOUTP_outputs] -> bus_selector23/1
  Ground2/1 -> FUSIONSWVar1/1(FUSIONSWVar1)
  Ground3/1 -> FUSIONSWVar2/1(FUSIONSWVar2)
  Ground4/1 -> FUSIONSWVar3/1(FUSIONSWVar3)
  Ground5/1 -> FUSIONSWVar4/1(FUSIONSWVar4)
  Ground6/1 -> FUSIONSWVar5/1(FUSIONSWVar5)
  bus_selector24/1 -> FUSIONSWchange1/1(FUSIONSWchange1)  "<VOUTP_Change1_cnt>"
  [BOUTP_outputs] -> bus_selector24/1
  bus_selector25/1 -> FUSIONSWchange2/1(FUSIONSWchange2)  "<VOUTP_Change2_cnt>"
  [BOUTP_outputs] -> bus_selector25/1
  bus_selector26/1 -> FUSIONSWdash1/1(FUSIONSWdash1)  "<VOUTP_Dash1_cnt>"
  [BOUTP_outputs] -> bus_selector26/1
  bus_selector27/1 -> FUSIONSWdash2/1(FUSIONSWdash2)  "<VOUTP_Dash2_cnt>"
  [BOUTP_outputs] -> bus_selector27/1

== system halout/HAL_OUT/CAN2/GW2_C10_0_0x1B3 ==
  BSCP_outputs : Inport  OutDataTypeStr=Bus: BSCP_outputs
  BOUTP_outputs : Inport  Port=2  OutDataTypeStr=Bus: BOUTP_outputs
  ABSActive : Subsystem
  ABSFailed : Subsystem
  ABSWnlmpSta : Subsystem
  AVHFailed : Subsystem
  AmberWnlmpSta : Subsystem
  BrkSwSta : Subsystem
  Ground : Ground
  Ground1 : Ground
  HSAActive : Subsystem
  HSAFailed : Subsystem
  MeterIndVehSpeed : Subsystem
  RedWnlmpSta : Subsystem
  VehSpeed : Subsystem
  bus_creator : BusCreator  Inputs=11  OutDataTypeStr=Bus: DT_CAN2_SG_GW2_C10_0  NonVirtualBus=on
  bus_selector : BusSelector  OutputSignals=VOUTP_ABSActive_flg
  bus_selector1 : BusSelector  OutputSignals=VOUTP_ABSFailed_flg
  bus_selector2 : BusSelector  OutputSignals=VOUTP_ABSWnlmpSta_flg
  bus_selector3 : BusSelector  OutputSignals=VOUTP_AmberWnlmpSta_flg
  bus_selector4 : BusSelector  OutputSignals=VOUTP_SCPBrkSwSta_flg
  bus_selector5 : BusSelector  OutputSignals=VOUTP_HSAActive_flg
  bus_selector6 : BusSelector  OutputSignals=VOUTP_HSAFailed_flg
  bus_selector7 : BusSelector  OutputSignals=VOUTP_RedWnlmpSta_flg
  bus_selector8 : BusSelector  OutputSignals=VOUTP_Vehspeed_kph
  GW2_C10_0 : Outport
  wires:
  BSCP_outputs/1 -> [BSCP_outputs]
  BOUTP_outputs/1 -> [BOUTP_outputs]
  [CAN2_ABS_Active] -> bus_creator/1  "CAN2_ABS_Active"
  [CAN2_ABS_Failed] -> bus_creator/2  "CAN2_ABS_Failed"
  [CAN2_ABS_WnlmpSta] -> bus_creator/3  "CAN2_ABS_WnlmpSta"
  [CAN2_AVH_Failed] -> bus_creator/4  "CAN2_AVH_Failed"
  [CAN2_Amber_WnlmpSta] -> bus_creator/5  "CAN2_Amber_WnlmpSta"
  [CAN2_BrkSw_Sta] -> bus_creator/6  "CAN2_BrkSw_Sta"
  [CAN2_HSA_Active] -> bus_creator/7  "CAN2_HSA_Active"
  [CAN2_HSA_Failed] -> bus_creator/8  "CAN2_HSA_Failed"
  [CAN2_Meter_Ind_VehSpeed] -> bus_creator/9  "CAN2_Meter_Ind_VehSpeed"
  [CAN2_Red_WnlmpSta] -> bus_creator/10  "CAN2_Red_WnlmpSta"
  [CAN2_VehSpeed] -> bus_creator/11  "CAN2_VehSpeed"
  bus_creator/1 -> GW2_C10_0/1
  ABSActive/1(CAN2_ABS_Active) -> [CAN2_ABS_Active]
  ABSFailed/1(CAN2_ABS_Failed) -> [CAN2_ABS_Failed]
  ABSWnlmpSta/1(CAN2_ABS_WnlmpSta) -> [CAN2_ABS_WnlmpSta]
  AVHFailed/1(CAN2_AVH_Failed) -> [CAN2_AVH_Failed]
  AmberWnlmpSta/1(CAN2_Amber_WnlmpSta) -> [CAN2_Amber_WnlmpSta]
  BrkSwSta/1(CAN2_BrkSw_Sta) -> [CAN2_BrkSw_Sta]
  HSAActive/1(CAN2_HSA_Active) -> [CAN2_HSA_Active]
  HSAFailed/1(CAN2_HSA_Failed) -> [CAN2_HSA_Failed]
  MeterIndVehSpeed/1(CAN2_Meter_Ind_VehSpeed) -> [CAN2_Meter_Ind_VehSpeed]
  RedWnlmpSta/1(CAN2_Red_WnlmpSta) -> [CAN2_Red_WnlmpSta]
  VehSpeed/1(CAN2_VehSpeed) -> [CAN2_VehSpeed]
  bus_selector/1 -> ABSActive/1(ABSActive)  "<VOUTP_ABSActive_flg>"
  [BOUTP_outputs] -> bus_selector/1
  bus_selector1/1 -> ABSFailed/1(ABSFailed)  "<VOUTP_ABSFailed_flg>"
  [BOUTP_outputs] -> bus_selector1/1
  bus_selector2/1 -> ABSWnlmpSta/1(ABSWnlmpSta)  "<VOUTP_ABSWnlmpSta_flg>"
  [BOUTP_outputs] -> bus_selector2/1
  Ground/1 -> AVHFailed/1(AVHFailed)
  bus_selector3/1 -> AmberWnlmpSta/1(AmberWnlmpSta)  "<VOUTP_AmberWnlmpSta_flg>"
  [BOUTP_outputs] -> bus_selector3/1
  bus_selector4/1 -> BrkSwSta/1(BrkSwSta)  "<VOUTP_SCPBrkSwSta_flg>"
  [BOUTP_outputs] -> bus_selector4/1
  bus_selector5/1 -> HSAActive/1(HSAActive)  "<VOUTP_HSAActive_flg>"
  [BOUTP_outputs] -> bus_selector5/1
  bus_selector6/1 -> HSAFailed/1(HSAFailed)  "<VOUTP_HSAFailed_flg>"
  [BOUTP_outputs] -> bus_selector6/1
  Ground1/1 -> MeterIndVehSpeed/1(MeterIndVehSpeed)
  bus_selector7/1 -> RedWnlmpSta/1(RedWnlmpSta)  "<VOUTP_RedWnlmpSta_flg>"
  [BOUTP_outputs] -> bus_selector7/1
  bus_selector8/1 -> VehSpeed/1(VehSpeed)  "<VOUTP_Vehspeed_kph>"
  [BOUTP_outputs] -> bus_selector8/1

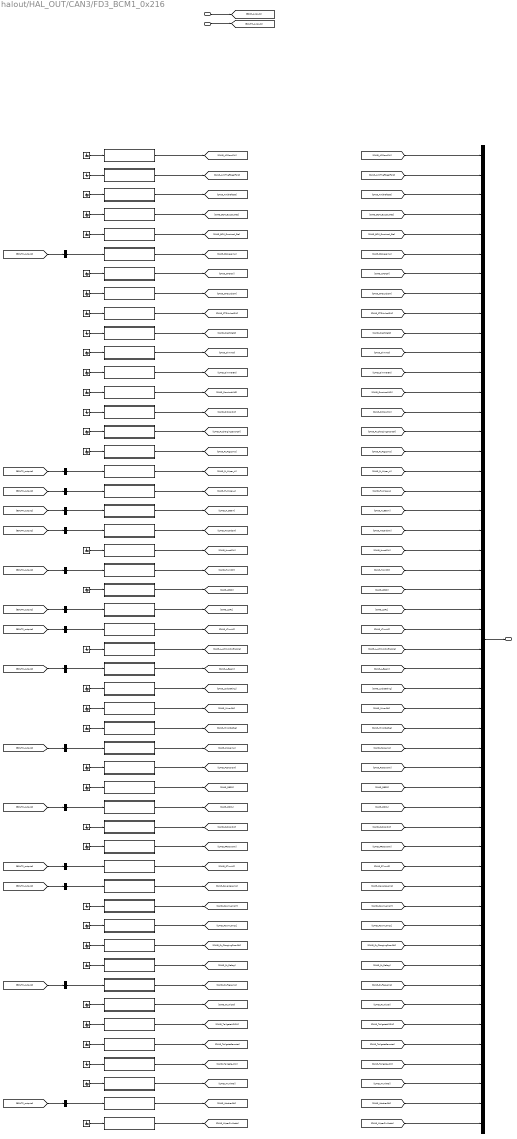
== system halout/HAL_OUT/CAN3/FD3_BCM1_0x216 ==
  BSCP_outputs : Inport  OutDataTypeStr=Bus: BSCP_outputs
  BOUTP_outputs : Inport  Port=2  OutDataTypeStr=Bus: BOUTP_outputs
  AllDoorSW : Subsystem
  AntiTheftSeatFold : Subsystem
  AntitheftSta : Subsystem
  BCMBuzzerReq : Subsystem
  BCMDoorLockSta : Subsystem
  BrakeLamp : Subsystem
  CTDCtrl : Subsystem
  CTDLockSW : Subsystem
  CTDUnlockSW : Subsystem
  CrashDetd : Subsystem
  Dimmer : Subsystem
  DimmerEN : Subsystem
  DoorLockIND : Subsystem
  DrDoorSW : Subsystem
  FrChargingDoorCtrl : Subsystem
  FrFogLamp : Subsystem
  FrWiperH : Subsystem
  FrWiperL : Subsystem
  Ground{,1..34} (35 alike) : Ground
  HBeam : Subsystem
  HazardSW : Subsystem
  HoodSW : Subsystem
  HornCtrl : Subsystem
  LAPMWdwEnable : Subsystem
  LBSD : Subsystem
  LBeam : Subsystem
  LDRL : Subsystem
  LTurnLP : Subsystem
  LockSetting : Subsystem
  MirrorCtrl : Subsystem
  MirrorDefog : Subsystem
  PosLamp : Subsystem
  PsDoorSW : Subsystem
  RBSD : Subsystem
  RDRL : Subsystem
  RLDoorSW : Subsystem
  RRDoorSW : Subsystem
  RTurnLP : Subsystem
  ReverseLamp : Subsystem
  RoomLampH : Subsystem
  RoomLampL : Subsystem
  RrChargingDoorCtrl : Subsystem
  RrDefog : Subsystem
  RrFogLamp : Subsystem
  RrWiper : Subsystem
  TailgateHDSW : Subsystem
  TailgateRemote : Subsystem
  TailgateSW : Subsystem
  TrunkRel : Subsystem
  WasherCtrl : Subsystem
  WiperFixMode : Subsystem
  bus_creator : BusCreator  Inputs=50  OutDataTypeStr=Bus: DT_CAN3_SG_FD3_BCM1  NonVirtualBus=on
  bus_selector : BusSelector  OutputSignals=VOUTP_BrakeLamp_flg
  bus_selector1 : BusSelector  OutputSignals=VOUTP_FrWiperH_flg
  bus_selector10 : BusSelector  OutputSignals=VOUTP_RDRL_flg
  bus_selector11 : BusSelector  OutputSignals=VOUTP_RTurnLP_flg
  bus_selector12 : BusSelector  OutputSignals=VOUTP_ReverseLamp_flg
  bus_selector13 : BusSelector  OutputSignals=VOUTP_RrFogLamp_flg
  bus_selector14 : BusSelector  OutputSignals=VOUTP_WasherCtrl_enum
  bus_selector2 : BusSelector  OutputSignals=VOUTP_FrWiperL_flg
  bus_selector3 : BusSelector  OutputSignals=VOUTP_HBeam_flg
  bus_selector4 : BusSelector  OutputSignals=VOUTP_HazardSW_flg
  bus_selector5 : BusSelector  OutputSignals=VOUTP_HornCtrl_flg
  bus_selector6 : BusSelector  OutputSignals=VOUTP_LDRL_flg
  bus_selector7 : BusSelector  OutputSignals=VOUTP_LTurnLP_flg
  bus_selector8 : BusSelector  OutputSignals=VOUTP_LBeam_flg
  bus_selector9 : BusSelector  OutputSignals=VOUTP_PosLamp_flg
  FD3_BCM1 : Outport
  wires:
  BSCP_outputs/1 -> [BSCP_outputs]
  BOUTP_outputs/1 -> [BOUTP_outputs]
  [CAN3_AllDoorSW] -> bus_creator/1  "CAN3_AllDoorSW"
  [CAN3_AntiTheftSeatFold] -> bus_creator/2  "CAN3_AntiTheftSeatFold"
  [CAN3_AntitheftSta] -> bus_creator/3  "CAN3_AntitheftSta"
  [CAN3_BCM_Buzzer_Req] -> bus_creator/4  "CAN3_BCM_Buzzer_Req"
  [CAN3_BCM_DoorLock_Sta] -> bus_creator/5  "CAN3_BCM_DoorLock_Sta"
  [CAN3_BrakeLamp] -> bus_creator/6  "CAN3_BrakeLamp"
  [CAN3_CTDCtrl] -> bus_creator/7  "CAN3_CTDCtrl"
  [CAN3_CTDLockSW] -> bus_creator/8  "CAN3_CTDLockSW"
  [CAN3_CTDUnlockSW] -> bus_creator/9  "CAN3_CTDUnlockSW"
  [CAN3_CrashDetd] -> bus_creator/10  "CAN3_CrashDetd"
  [CAN3_Dimmer] -> bus_creator/11  "CAN3_Dimmer"
  [CAN3_DimmerEN] -> bus_creator/12  "CAN3_DimmerEN"
  [CAN3_DoorLockIND] -> bus_creator/13  "CAN3_DoorLockIND"
  [CAN3_DrDoorSW] -> bus_creator/14  "CAN3_DrDoorSW"
  [CAN3_Fr_ChargingDoorCtrl] -> bus_creator/15  "CAN3_Fr_ChargingDoorCtrl"
  [CAN3_Fr_FogLamp] -> bus_creator/16  "CAN3_Fr_FogLamp"
  [CAN3_Fr_Wiper_H] -> bus_creator/17  "CAN3_Fr_Wiper_H"
  [CAN3_Fr_Wiper_L] -> bus_creator/18  "CAN3_Fr_Wiper_L"
  [CAN3_H_Beam] -> bus_creator/19  "CAN3_H_Beam"
  [CAN3_HazardSW] -> bus_creator/20  "CAN3_HazardSW"
  [CAN3_HoodSW] -> bus_creator/21  "CAN3_HoodSW"
  [CAN3_HornCtrl] -> bus_creator/22  "CAN3_HornCtrl"
  [CAN3_LBSD] -> bus_creator/23  "CAN3_LBSD"
  [CAN3_LDRL] -> bus_creator/24  "CAN3_LDRL"
  [CAN3_LTurnLP] -> bus_creator/25  "CAN3_LTurnLP"
  [CAN3_L_APM_WdwEnable] -> bus_creator/26  "CAN3_L_APM_WdwEnable"
  [CAN3_L_Beam] -> bus_creator/27  "CAN3_L_Beam"
  [CAN3_LockSetting] -> bus_creator/28  "CAN3_LockSetting"
  [CAN3_MirrorCtrl] -> bus_creator/29  "CAN3_MirrorCtrl"
  [CAN3_MirrorDefog] -> bus_creator/30  "CAN3_MirrorDefog"
  [CAN3_PosLamp] -> bus_creator/31  "CAN3_PosLamp"
  [CAN3_PsDoorSW] -> bus_creator/32  "CAN3_PsDoorSW"
  [CAN3_RBSD] -> bus_creator/33  "CAN3_RBSD"
  [CAN3_RDRL] -> bus_creator/34  "CAN3_RDRL"
  [CAN3_RLDoorSW] -> bus_creator/35  "CAN3_RLDoorSW"
  [CAN3_RRDoorSW] -> bus_creator/36  "CAN3_RRDoorSW"
  [CAN3_RTurnLP] -> bus_creator/37  "CAN3_RTurnLP"
  [CAN3_ReverseLamp] -> bus_creator/38  "CAN3_ReverseLamp"
  [CAN3_RoomLampH] -> bus_creator/39  "CAN3_RoomLampH"
  [CAN3_RoomLampL] -> bus_creator/40  "CAN3_RoomLampL"
  [CAN3_Rr_ChargingDoorCtrl] -> bus_creator/41  "CAN3_Rr_ChargingDoorCtrl"
  [CAN3_Rr_Defog] -> bus_creator/42  "CAN3_Rr_Defog"
  [CAN3_Rr_FogLamp] -> bus_creator/43  "CAN3_Rr_FogLamp"
  [CAN3_Rr_Wiper] -> bus_creator/44  "CAN3_Rr_Wiper"
  [CAN3_TailgateHDSW] -> bus_creator/45  "CAN3_TailgateHDSW"
  [CAN3_TailgateRemote] -> bus_creator/46  "CAN3_TailgateRemote"
  [CAN3_Tailgate_SW] -> bus_creator/47  "CAN3_Tailgate_SW"
  [CAN3_TrunkRel] -> bus_creator/48  "CAN3_TrunkRel"
  [CAN3_WasherCtrl] -> bus_creator/49  "CAN3_WasherCtrl"
  [CAN3_WiperFixMode] -> bus_creator/50  "CAN3_WiperFixMode"
  bus_creator/1 -> FD3_BCM1/1
  AllDoorSW/1(CAN3_AllDoorSW) -> [CAN3_AllDoorSW]
  AntiTheftSeatFold/1(CAN3_AntiTheftSeatFold) -> [CAN3_AntiTheftSeatFold]
  AntitheftSta/1(CAN3_AntitheftSta) -> [CAN3_AntitheftSta]
  BCMBuzzerReq/1(CAN3_BCM_Buzzer_Req) -> [CAN3_BCM_Buzzer_Req]
  BCMDoorLockSta/1(CAN3_BCM_DoorLock_Sta) -> [CAN3_BCM_DoorLock_Sta]
  BrakeLamp/1(CAN3_BrakeLamp) -> [CAN3_BrakeLamp]
  CTDCtrl/1(CAN3_CTDCtrl) -> [CAN3_CTDCtrl]
  CTDLockSW/1(CAN3_CTDLockSW) -> [CAN3_CTDLockSW]
  CTDUnlockSW/1(CAN3_CTDUnlockSW) -> [CAN3_CTDUnlockSW]
  CrashDetd/1(CAN3_CrashDetd) -> [CAN3_CrashDetd]
  Dimmer/1(CAN3_Dimmer) -> [CAN3_Dimmer]
  DimmerEN/1(CAN3_DimmerEN) -> [CAN3_DimmerEN]
  DoorLockIND/1(CAN3_DoorLockIND) -> [CAN3_DoorLockIND]
  DrDoorSW/1(CAN3_DrDoorSW) -> [CAN3_DrDoorSW]
  FrChargingDoorCtrl/1(CAN3_Fr_ChargingDoorCtrl) -> [CAN3_Fr_ChargingDoorCtrl]
  FrFogLamp/1(CAN3_Fr_FogLamp) -> [CAN3_Fr_FogLamp]
  FrWiperH/1(CAN3_Fr_Wiper_H) -> [CAN3_Fr_Wiper_H]
  FrWiperL/1(CAN3_Fr_Wiper_L) -> [CAN3_Fr_Wiper_L]
  HBeam/1(CAN3_H_Beam) -> [CAN3_H_Beam]
  HazardSW/1(CAN3_HazardSW) -> [CAN3_HazardSW]
  HoodSW/1(CAN3_HoodSW) -> [CAN3_HoodSW]
  HornCtrl/1(CAN3_HornCtrl) -> [CAN3_HornCtrl]
  LBSD/1(CAN3_LBSD) -> [CAN3_LBSD]
  LDRL/1(CAN3_LDRL) -> [CAN3_LDRL]
  LTurnLP/1(CAN3_LTurnLP) -> [CAN3_LTurnLP]
  LAPMWdwEnable/1(CAN3_L_APM_WdwEnable) -> [CAN3_L_APM_WdwEnable]
  LBeam/1(CAN3_L_Beam) -> [CAN3_L_Beam]
  LockSetting/1(CAN3_LockSetting) -> [CAN3_LockSetting]
  MirrorCtrl/1(CAN3_MirrorCtrl) -> [CAN3_MirrorCtrl]
  MirrorDefog/1(CAN3_MirrorDefog) -> [CAN3_MirrorDefog]
  PosLamp/1(CAN3_PosLamp) -> [CAN3_PosLamp]
  PsDoorSW/1(CAN3_PsDoorSW) -> [CAN3_PsDoorSW]
  RBSD/1(CAN3_RBSD) -> [CAN3_RBSD]
  RDRL/1(CAN3_RDRL) -> [CAN3_RDRL]
  RLDoorSW/1(CAN3_RLDoorSW) -> [CAN3_RLDoorSW]
  RRDoorSW/1(CAN3_RRDoorSW) -> [CAN3_RRDoorSW]
  RTurnLP/1(CAN3_RTurnLP) -> [CAN3_RTurnLP]
  ReverseLamp/1(CAN3_ReverseLamp) -> [CAN3_ReverseLamp]
  RoomLampH/1(CAN3_RoomLampH) -> [CAN3_RoomLampH]
  RoomLampL/1(CAN3_RoomLampL) -> [CAN3_RoomLampL]
  RrChargingDoorCtrl/1(CAN3_Rr_ChargingDoorCtrl) -> [CAN3_Rr_ChargingDoorCtrl]
  RrDefog/1(CAN3_Rr_Defog) -> [CAN3_Rr_Defog]
  RrFogLamp/1(CAN3_Rr_FogLamp) -> [CAN3_Rr_FogLamp]
  RrWiper/1(CAN3_Rr_Wiper) -> [CAN3_Rr_Wiper]
  TailgateHDSW/1(CAN3_TailgateHDSW) -> [CAN3_TailgateHDSW]
  TailgateRemote/1(CAN3_TailgateRemote) -> [CAN3_TailgateRemote]
  TailgateSW/1(CAN3_Tailgate_SW) -> [CAN3_Tailgate_SW]
  TrunkRel/1(CAN3_TrunkRel) -> [CAN3_TrunkRel]
  WasherCtrl/1(CAN3_WasherCtrl) -> [CAN3_WasherCtrl]
  WiperFixMode/1(CAN3_WiperFixMode) -> [CAN3_WiperFixMode]
  Ground/1 -> AllDoorSW/1(AllDoorSW)
  Ground1/1 -> AntiTheftSeatFold/1(AntiTheftSeatFold)
  Ground2/1 -> AntitheftSta/1(AntitheftSta)
  Ground3/1 -> BCMBuzzerReq/1(BCMBuzzerReq)
  Ground4/1 -> BCMDoorLockSta/1(BCMDoorLockSta)
  bus_selector/1 -> BrakeLamp/1(BrakeLamp)  "<VOUTP_BrakeLamp_flg>"
  [BOUTP_outputs] -> bus_selector/1
  Ground5/1 -> CTDCtrl/1(CTDCtrl)
  Ground6/1 -> CTDLockSW/1(CTDLockSW)
  Ground7/1 -> CTDUnlockSW/1(CTDUnlockSW)
  Ground8/1 -> CrashDetd/1(CrashDetd)
  Ground9/1 -> Dimmer/1(Dimmer)
  Ground10/1 -> DimmerEN/1(DimmerEN)
  Ground11/1 -> DoorLockIND/1(DoorLockIND)
  Ground12/1 -> DrDoorSW/1(DrDoorSW)
  Ground13/1 -> FrChargingDoorCtrl/1(FrChargingDoorCtrl)
  Ground14/1 -> FrFogLamp/1(FrFogLamp)
  bus_selector1/1 -> FrWiperH/1(FrWiperH)  "<VOUTP_FrWiperH_flg>"
  [BOUTP_outputs] -> bus_selector1/1
  bus_selector2/1 -> FrWiperL/1(FrWiperL)  "<VOUTP_FrWiperL_flg>"
  [BOUTP_outputs] -> bus_selector2/1
  bus_selector3/1 -> HBeam/1(HBeam)  "<VOUTP_HBeam_flg>"
  [BOUTP_outputs] -> bus_selector3/1
  bus_selector4/1 -> HazardSW/1(HazardSW)  "<VOUTP_HazardSW_flg>"
  [BOUTP_outputs] -> bus_selector4/1
  Ground15/1 -> HoodSW/1(HoodSW)
  bus_selector5/1 -> HornCtrl/1(HornCtrl)  "<VOUTP_HornCtrl_flg>"
  [BOUTP_outputs] -> bus_selector5/1
  Ground16/1 -> LBSD/1(LBSD)
  bus_selector6/1 -> LDRL/1(LDRL)  "<VOUTP_LDRL_flg>"
  [BOUTP_outputs] -> bus_selector6/1
  bus_selector7/1 -> LTurnLP/1(LTurnLP)  "<VOUTP_LTurnLP_flg>"
  [BOUTP_outputs] -> bus_selector7/1
  Ground17/1 -> LAPMWdwEnable/1(LAPMWdwEnable)
  bus_selector8/1 -> LBeam/1(LBeam)  "<VOUTP_LBeam_flg>"
  [BOUTP_outputs] -> bus_selector8/1
  Ground18/1 -> LockSetting/1(LockSetting)
  Ground19/1 -> MirrorCtrl/1(MirrorCtrl)
  Ground20/1 -> MirrorDefog/1(MirrorDefog)
  bus_selector9/1 -> PosLamp/1(PosLamp)  "<VOUTP_PosLamp_flg>"
  [BOUTP_outputs] -> bus_selector9/1
  Ground21/1 -> PsDoorSW/1(PsDoorSW)
  Ground22/1 -> RBSD/1(RBSD)
  bus_selector10/1 -> RDRL/1(RDRL)  "<VOUTP_RDRL_flg>"
  [BOUTP_outputs] -> bus_selector10/1
  Ground23/1 -> RLDoorSW/1(RLDoorSW)
  Ground24/1 -> RRDoorSW/1(RRDoorSW)
  bus_selector11/1 -> RTurnLP/1(RTurnLP)  "<VOUTP_RTurnLP_flg>"
  [BOUTP_outputs] -> bus_selector11/1
  bus_selector12/1 -> ReverseLamp/1(ReverseLamp)  "<VOUTP_ReverseLamp_flg>"
  [BOUTP_outputs] -> bus_selector12/1
  Ground25/1 -> RoomLampH/1(RoomLampH)
  Ground26/1 -> RoomLampL/1(RoomLampL)
  Ground27/1 -> RrChargingDoorCtrl/1(RrChargingDoorCtrl)
  Ground28/1 -> RrDefog/1(RrDefog)
  bus_selector13/1 -> RrFogLamp/1(RrFogLamp)  "<VOUTP_RrFogLamp_flg>"
  [BOUTP_outputs] -> bus_selector13/1
  Ground29/1 -> RrWiper/1(RrWiper)
  Ground30/1 -> TailgateHDSW/1(TailgateHDSW)
  Ground31/1 -> TailgateRemote/1(TailgateRemote)
  Ground32/1 -> TailgateSW/1(TailgateSW)
  Ground33/1 -> TrunkRel/1(TrunkRel)
  bus_selector14/1 -> WasherCtrl/1(WasherCtrl)  "<VOUTP_WasherCtrl_enum>"
  [BOUTP_outputs] -> bus_selector14/1
  Ground34/1 -> WiperFixMode/1(WiperFixMode)
